simulink model "switching_controller_parallel_after_retraining"  (R2020a)
settings: Solver=FixedStepAuto  StartTime=0.0  StopTime=simulation.time_window  FixedStep=simulation.time_step  MaxStep=.2  RelTol=1e-3
model workspace (MAT data in the model file):
  PID_TRESH = 0.3
undefined symbols (not defined in the file): DiscIntNeverNeededParam
libraries: neural x72, simulink x1
(part 3 of 3)

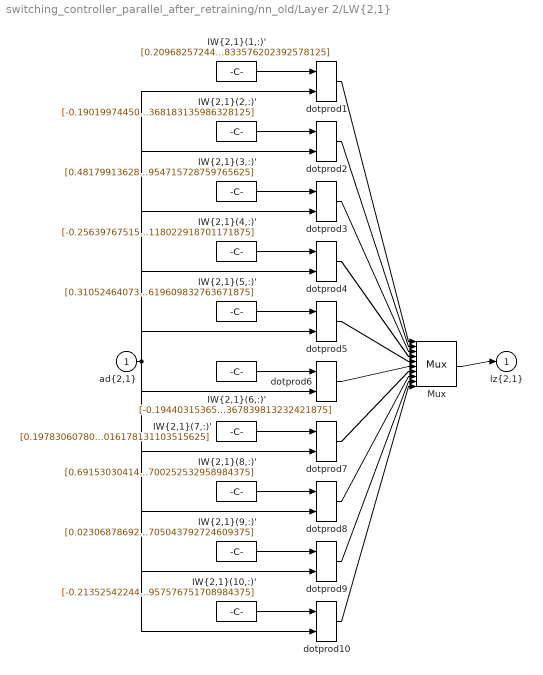
== system switching_controller_parallel_after_retraining/nn_old/Layer 2/LW{2,1} ==
  "ad{2,1}" : Inport  PortDimensions=20
      mask Display: e = 0.06;c1 = [120 230 180]/255;c2 = ([120 230 180]+0)/(256+128);c3 = ([120 230 180]+128)/(256+128);patch([0 1 1 0],[0 0 1 1],c1);patch([0 1 1 1-e 1-e 0+e],[0 0 1 1-e 0+e 0+e],c2);patch([0 0 1 1-e 0+e 0+e],[0 1 1 1-e 1-e 0+e],c3);plot([0 1 1 0 0],[0 0 1 1 0]);
  "IW{2,1}(1,:)'" : Constant  Value=[0.2096825724481717612146525198113522492349147796630859375;-0.0786324900654914726860766904792399145662784576416015625;-0.437914448078958240540003998830798082053661346435546875;0.1697961511740600226705311115438234992325305938720703125;0.55023489427883287561371616902761161327362060546875;-0.264125067565491977727987205071258358657360076904296875;-0.51948962376459417722429634522995911538600921630859375;0.332243447773037214876268308216822333633899688720703125;0.1565170256116675540081217832266702316701412200927734375;-0.63070597920798121549523784779012203216552734375;-0.27205863960363274589582260887254960834980010986328125;-0.1899107392996790821815267236161162145435810089111328125;-0.1897375152263709174871308960064197890460491180419921875;0.0256999070051998797226122661641056765802204608917236328125;0.309106789683368965437892939007724635303020477294921875;0.41159516280277974598078571943915449082851409912109375;0.394189668439436535773978675933904014527797698974609375;-0.58049288962487277654389572489890269935131072998046875;-0.3828300990267410330858410816290415823459625244140625;0.107169998780845709962505907242302782833576202392578125]
      mask Display: e = 0.06;c1 = [120 150 230]/255;c2 = ([120 150 230]+0)/383;c3 = ([120 150 230]+128)/383;patch([0 1 1 0],[0 0 1 1],c1);patch([0 1 1 1-e 1-e 0+e],[0 0 1 1-e 0+e 0+e],c2);patch([0 0 1 1-e 0+e 0+e],[0 1 1 1-e 1-e 0+e],c3);plot([0 1 1 0 0],[0 0 1 1 0]);disp('weights');
  "IW{2,1}(10,:)'" : Constant  Value=[-0.2135254224475679196704192008837708272039890289306640625;-0.46702854909986057929671687816153280436992645263671875;-0.491012465365010697393444161207298748195171356201171875;-0.56496432763406811972117793629877269268035888671875;-0.7227133704126142976775781789910979568958282470703125;0.170979606044271481568586068533477373421192169189453125;0.44374389503406319601452878487179987132549285888671875;0.0753589669229797476379673071278375573456287384033203125;-0.451293781769779134283027133278665132820606231689453125;0.0747381398083216963446062663933844305574893951416015625;-0.2762075487214932234536490796017460525035858154296875;-0.5460267148614048604571280520758591592311859130859375;0.0197077459717405478745178015742567367851734161376953125;-0.06834329138225274380413765129560488276183605194091796875;-0.1274719116559372700248076171192224137485027313232421875;-0.2139125442383393582712614033880527131259441375732421875;0.08760130810873280327033540970660396851599216461181640625;-0.10338035652578873857532215652099694125354290008544921875;0.2862039857027902645114636470680125057697296142578125;0.207128935024094518180248769567697308957576751708984375]
      mask Display: e = 0.06;c1 = [120 150 230]/255;c2 = ([120 150 230]+0)/383;c3 = ([120 150 230]+128)/383;patch([0 1 1 0],[0 0 1 1],c1);patch([0 1 1 1-e 1-e 0+e],[0 0 1 1-e 0+e 0+e],c2);patch([0 0 1 1-e 0+e 0+e],[0 1 1 1-e 1-e 0+e],c3);plot([0 1 1 0 0],[0 0 1 1 0]);disp('weights');
  "IW{2,1}(2,:)'" : Constant  Value=[-0.1901997445055658986223789952418883331120014190673828125;0.4889226492339562302191779963322915136814117431640625;0.5822125104488617974851649705669842660427093505859375;0.04192611403211977949556654721163795329630374908447265625;-0.068996957352157384235624704160727560520172119140625;-0.433158542617962993848124142459710128605365753173828125;-0.040131359594994149564417540432259556837379932403564453125;0.1937276670045855464508122167899273335933685302734375;0.452152014649461919670869747278629802167415618896484375;-0.55286960480626989866692611030885018408298492431640625;0.08355940035194704684773370217953925020992755889892578125;-0.1743526015010171958952156501254648901522159576416015625;0.11476795054229714521110139457960030995309352874755859375;-0.59479734978772358378051876570680178701877593994140625;0.276319293859086323461582423988147638738155364990234375;-0.10215476488676560051782615801130305044353008270263671875;-0.26107272028639816330297662716475315392017364501953125;-0.579920390991560896765122379292733967304229736328125;-0.1592627650723278665001458875849493779242038726806640625;-0.044346946533229077147542085413078893907368183135986328125]
      mask Display: e = 0.06;c1 = [120 150 230]/255;c2 = ([120 150 230]+0)/383;c3 = ([120 150 230]+128)/383;patch([0 1 1 0],[0 0 1 1],c1);patch([0 1 1 1-e 1-e 0+e],[0 0 1 1-e 0+e 0+e],c2);patch([0 0 1 1-e 0+e 0+e],[0 1 1 1-e 1-e 0+e],c3);plot([0 1 1 0 0],[0 0 1 1 0]);disp('weights');
  "IW{2,1}(3,:)'" : Constant  Value=[0.481799136287025364655534076518961228430271148681640625;0.387006958211107809919582223301404155790805816650390625;0.1919190370005954549004201226125587709248065948486328125;-0.43641483886599996555588631963473744690418243408203125;-0.49688357411208039504657563156797550618648529052734375;0.0020488012679514230364452576083067469880916178226470947265625;-0.184908572502721690877791616003378294408321380615234375;0.333455839511515084172543765816953964531421661376953125;-0.481036487364089826446189590569701977074146270751953125;0.34755666012205954640279514933354221284389495849609375;0.294843116199611898764487705193459987640380859375;0.2329942803063660139439861040955292992293834686279296875;-0.332425721969732690386223339373827911913394927978515625;-0.11204195263561367301718973976676352322101593017578125;-0.064344226389462966242405173034057952463626861572265625;-0.26447918257127212005030969521612860262393951416015625;-0.4404023331890851711278855873388238251209259033203125;-0.43485200204655460876068673314875923097133636474609375;0.4669108714352014910531352143152616918087005615234375;-0.387250838515266926354030374568537808954715728759765625]
      mask Display: e = 0.06;c1 = [120 150 230]/255;c2 = ([120 150 230]+0)/383;c3 = ([120 150 230]+128)/383;patch([0 1 1 0],[0 0 1 1],c1);patch([0 1 1 1-e 1-e 0+e],[0 0 1 1-e 0+e 0+e],c2);patch([0 0 1 1-e 0+e 0+e],[0 1 1 1-e 1-e 0+e],c3);plot([0 1 1 0 0],[0 0 1 1 0]);disp('weights');
  "IW{2,1}(4,:)'" : Constant  Value=[-0.25639767515399736197423408157192170619964599609375;-0.45921838490317312686528339327196590602397918701171875;-0.3293254038638953051787439108011312782764434814453125;-0.44158108947889973538991625900962390005588531494140625;0.233955749562186399170826689442037604749202728271484375;-0.027814737908238289232354389923784765414893627166748046875;-0.880326454366271438090052470215596258640289306640625;-0.1700238043081334915473945557096158154308795928955078125;-0.260201087444173750906628583834390155971050262451171875;0.52249104272064117449048126218258403241634368896484375;-0.045211937144701015711678593333999742753803730010986328125;0.056005248738155342935751690447432338260114192962646484375;0.0272144426463411977235029581834169221110641956329345703125;-0.55189260887602886729297324563958682119846343994140625;-0.2232599587265805818336872334839426912367343902587890625;-0.77589840738633253369727071913075633347034454345703125;-0.364528533738595894586609347243211232125759124755859375;-0.52690429597504129244356363415136002004146575927734375;0.2355191475436664294562660870724357664585113525390625;0.1088197708787270456820550634802202694118022918701171875]
      mask Display: e = 0.06;c1 = [120 150 230]/255;c2 = ([120 150 230]+0)/383;c3 = ([120 150 230]+128)/383;patch([0 1 1 0],[0 0 1 1],c1);patch([0 1 1 1-e 1-e 0+e],[0 0 1 1-e 0+e 0+e],c2);patch([0 0 1 1-e 0+e 0+e],[0 1 1 1-e 1-e 0+e],c3);plot([0 1 1 0 0],[0 0 1 1 0]);disp('weights');
  "IW{2,1}(5,:)'" : Constant  Value=[0.310524640737501023135536115660215727984905242919921875;0.0146429681645852023674780895134972524829208850860595703125;0.416071005130671578431389434626908041536808013916015625;0.2349476910365399240365746891257003881037235260009765625;0.0266711848666466681823106199544781702570617198944091796875;-0.2184710102237388540391549440755625255405902862548828125;2.094726675060243348269750640611164271831512451171875;-0.62331361106756000278750207144184969365596771240234375;-0.0203637098643958715238344581166529678739607334136962890625;-0.0271757616677543722971677198074758052825927734375;-0.099119675867250067735625407294719479978084564208984375;0.12043446514574361605465213642673916183412075042724609375;-0.88670130489474974222474656926351599395275115966796875;0.25211544537308194779967607246362604200839996337890625;-0.11259143114996773837876986590345040895044803619384765625;0.61060143798205601672890452391584403812885284423828125;-0.452607547304984703107066934535396285355091094970703125;-0.373800814753432908421615366023615933954715728759765625;-0.0172484013592278662141410450203693471848964691162109375;0.5859028956126166587381476347218267619609832763671875]
      mask Display: e = 0.06;c1 = [120 150 230]/255;c2 = ([120 150 230]+0)/383;c3 = ([120 150 230]+128)/383;patch([0 1 1 0],[0 0 1 1],c1);patch([0 1 1 1-e 1-e 0+e],[0 0 1 1-e 0+e 0+e],c2);patch([0 0 1 1-e 0+e 0+e],[0 1 1 1-e 1-e 0+e],c3);plot([0 1 1 0 0],[0 0 1 1 0]);disp('weights');
  "IW{2,1}(6,:)'" : Constant  Value=[-0.1944031536556706518670267769266502000391483306884765625;-0.295446194500971426322166735189966857433319091796875;-0.54770988104943951757519471357227303087711334228515625;-0.404408826705410950896890653893933631479740142822265625;-0.83869791765557566431965597075759433209896087646484375;-0.325816969167355974246191863130661658942699432373046875;-0.2072529611842870156390716829264420084655284881591796875;0.240744674786417700573792899376712739467620849609375;-0.1674498692919050568672645340484450571238994598388671875;-0.28891816291228311630590042113908566534519195556640625;-0.22131051344031948957535860245116055011749267578125;-0.10913280135527003711359839144279249012470245361328125;-0.4918651471215065296149759888066910207271575927734375;0.240001755562789742537432857716339640319347381591796875;0.6937710080396275458269883529283106327056884765625;0.06323702674474794560577350921448669396340847015380859375;-0.2752337038543775094012744375504553318023681640625;-0.255069800974772997737005653107189573347568511962890625;-0.285682618796993192944455586257390677928924560546875;-0.31188153451426436912896633657510392367839813232421875]
      mask Display: e = 0.06;c1 = [120 150 230]/255;c2 = ([120 150 230]+0)/383;c3 = ([120 150 230]+128)/383;patch([0 1 1 0],[0 0 1 1],c1);patch([0 1 1 1-e 1-e 0+e],[0 0 1 1-e 0+e 0+e],c2);patch([0 0 1 1-e 0+e 0+e],[0 1 1 1-e 1-e 0+e],c3);plot([0 1 1 0 0],[0 0 1 1 0]);disp('weights');
  "IW{2,1}(7,:)'" : Constant  Value=[0.1978306078065260875664677087115705944597721099853515625;-0.59250058903084179551257193452329374849796295166015625;0.64639267817649359582077295272029004991054534912109375;-0.53285927855746084702559528523124754428863525390625;0.588817119499761343348609443637542426586151123046875;-0.348911668719428025298157081124372780323028564453125;-0.64457560060689800263133975022356025874614715576171875;0.0562679680258353076549582283405470661818981170654296875;0.5623436544941402548403175387647934257984161376953125;0.1281096810622278925340111754849203862249851226806640625;0.161634591264916249730987374277901835739612579345703125;-0.313017483079470526519116901909001171588897705078125;0.38128996525822411722828064739587716758251190185546875;-0.1756877707290915580085055580639163963496685028076171875;-0.380091610378465116770740905849379487335681915283203125;-0.1356942844701036487986556267060223035514354705810546875;0.1185198788428162564034806791823939420282840728759765625;-0.254421588692579081492084469573455862700939178466796875;-0.2881679500781364478001478346413932740688323974609375;-0.2391992576729999042672858422520221211016178131103515625]
      mask Display: e = 0.06;c1 = [120 150 230]/255;c2 = ([120 150 230]+0)/383;c3 = ([120 150 230]+128)/383;patch([0 1 1 0],[0 0 1 1],c1);patch([0 1 1 1-e 1-e 0+e],[0 0 1 1-e 0+e 0+e],c2);patch([0 0 1 1-e 0+e 0+e],[0 1 1 1-e 1-e 0+e],c3);plot([0 1 1 0 0],[0 0 1 1 0]);disp('weights');
  "IW{2,1}(8,:)'" : Constant  Value=[0.6915303041485005852706535733886994421482086181640625;-0.013943214076003206114418020433731726370751857757568359375;0.197633492735798832473648189989035017788410186767578125;-0.1829294585786688520645526523367152549326419830322265625;0.41194460235457064367636803581262938678264617919921875;0.2697850457965962345241450748289935290813446044921875;0.2278285465289087985407689984640455804765224456787109375;-0.594187771563595479307196001172997057437896728515625;0.33636923738323110111281266654259525239467620849609375;-0.10886422192579021939184968914560158737003803253173828125;0.330016039728184329415938691454357467591762542724609375;-0.5612454717224470979175521279103122651576995849609375;-0.5208533730307125519942701430409215390682220458984375;0.0927595999828694228739323079935275018215179443359375;-0.295470908532163789583790958204190246760845184326171875;0.2464488470485728111025736097872140817344188690185546875;-0.253925461039385014228031423044740222394466400146484375;-0.44676839807914936475441436414257623255252838134765625;-0.343537111312336163049252490964136086404323577880859375;0.04503529300945828539592952211023657582700252532958984375]
      mask Display: e = 0.06;c1 = [120 150 230]/255;c2 = ([120 150 230]+0)/383;c3 = ([120 150 230]+128)/383;patch([0 1 1 0],[0 0 1 1],c1);patch([0 1 1 1-e 1-e 0+e],[0 0 1 1-e 0+e 0+e],c2);patch([0 0 1 1-e 0+e 0+e],[0 1 1 1-e 1-e 0+e],c3);plot([0 1 1 0 0],[0 0 1 1 0]);disp('weights');
  "IW{2,1}(9,:)'" : Constant  Value=[0.0230687869274933711472019837174229905940592288970947265625;0.063142758058253922737179664181894622743129730224609375;0.15173098751753089086236059301882050931453704833984375;0.00443276217291526698771608749893857748247683048248291015625;0.3879819604221512729935739116626791656017303466796875;0.67423681207509444934800058035762049257755279541015625;-0.10965154605191219927551316004610271193087100982666015625;0.54284957310125514506893296129419468343257904052734375;0.485695834032557727244494572005351074039936065673828125;-0.3061948412592043755608983701677061617374420166015625;0.359525507608165872941441421062336303293704986572265625;0.60766075733581847995168345732963643968105316162109375;-0.1918328188570195547146823855655384249985218048095703125;0.56745984668721305421712486349861137568950653076171875;0.392602621322820033444855880588875152170658111572265625;-0.534358634420198708170346435508690774440765380859375;0.023661369862847399236915890696764108724892139434814453125;-0.1696865058591041364177698369530844502151012420654296875;0.4660595474214745959073979975073598325252532958984375;-0.439829607094486652041354091124958358705043792724609375]
      mask Display: e = 0.06;c1 = [120 150 230]/255;c2 = ([120 150 230]+0)/383;c3 = ([120 150 230]+128)/383;patch([0 1 1 0],[0 0 1 1],c1);patch([0 1 1 1-e 1-e 0+e],[0 0 1 1-e 0+e 0+e],c2);patch([0 0 1 1-e 0+e 0+e],[0 1 1 1-e 1-e 0+e],c3);plot([0 1 1 0 0],[0 0 1 1 0]);disp('weights');
  Mux : Mux  Inputs=10
      mask Display: e = 0.06;c1 = [120 150 230]/255;c2 = ([120 150 230]+0)/383;c3 = ([120 150 230]+128)/383;patch([0 1 1 0],[0 0 1 1],c1);patch([0 1 1 1-e 1-e 0+e],[0 0 1 1-e 0+e 0+e],c2);patch([0 0 1 1-e 0+e 0+e],[0 1 1 1-e 1-e 0+e],c3);plot([0 1 1 0 0],[0 0 1 1 0]);disp('Mux');
  dotprod{1..10} (10 alike) : neural/Weight Functions/dotprod
  "lz{2,1}" : Outport
      mask Display: e = 0.06;c1 = [120 230 180]/255;c2 = ([120 230 180]+0)/(256+128);c3 = ([120 230 180]+128)/(256+128);patch([0 1 1 0],[0 0 1 1],c1);patch([0 1 1 1-e 1-e 0+e],[0 0 1 1-e 0+e 0+e],c2);patch([0 0 1 1-e 0+e 0+e],[0 1 1 1-e 1-e 0+e],c3);plot([0 1 1 0 0],[0 0 1 1 0]);
  wires:
  "IW{2,1}(1,:)'"/1 -> dotprod1/1
  "ad{2,1}"/1 -> dotprod1/2, dotprod2/2, dotprod3/2, dotprod4/2, dotprod5/2, dotprod6/2, dotprod7/2, dotprod8/2, dotprod9/2, dotprod10/2
  dotprod1/1 -> Mux/1
  "IW{2,1}(2,:)'"/1 -> dotprod2/1
  dotprod2/1 -> Mux/2
  "IW{2,1}(3,:)'"/1 -> dotprod3/1
  dotprod3/1 -> Mux/3
  "IW{2,1}(4,:)'"/1 -> dotprod4/1
  dotprod4/1 -> Mux/4
  "IW{2,1}(5,:)'"/1 -> dotprod5/1
  dotprod5/1 -> Mux/5
  "IW{2,1}(6,:)'"/1 -> dotprod6/1
  dotprod6/1 -> Mux/6
  "IW{2,1}(7,:)'"/1 -> dotprod7/1
  dotprod7/1 -> Mux/7
  "IW{2,1}(8,:)'"/1 -> dotprod8/1
  dotprod8/1 -> Mux/8
  "IW{2,1}(9,:)'"/1 -> dotprod9/1
  dotprod9/1 -> Mux/9
  "IW{2,1}(10,:)'"/1 -> dotprod10/1
  dotprod10/1 -> Mux/10
  Mux/1 -> "lz{2,1}"/1

== system switching_controller_parallel_after_retraining/nn_old/Layer 3/Delays 1 ==
  "p{3}" : Inport  PortDimensions=10
      mask Display: e = 0.06;c1 = [120 230 180]/255;c2 = ([120 230 180]+0)/(256+128);c3 = ([120 230 180]+128)/(256+128);patch([0 1 1 0],[0 0 1 1],c1);patch([0 1 1 1-e 1-e 0+e],[0 0 1 1-e 0+e 0+e],c2);patch([0 0 1 1-e 0+e 0+e],[0 1 1 1-e 1-e 0+e],c3);plot([0 1 1 0 0],[0 0 1 1 0]);
  mux : Mux  Inputs=1
      mask Display: e = 0.06;c1 = [120 150 230]/255;c2 = ([120 150 230]+0)/383;c3 = ([120 150 230]+128)/383;patch([0 1 1 0],[0 0 1 1],c1);patch([0 1 1 1-e 1-e 0+e],[0 0 1 1-e 0+e 0+e],c2);patch([0 0 1 1-e 0+e 0+e],[0 1 1 1-e 1-e 0+e],c3);plot([0 1 1 0 0],[0 0 1 1 0]);disp('Mux')
  "pd{3,2}" : Outport
      mask Display: e = 0.06;c1 = [120 230 180]/255;c2 = ([120 230 180]+0)/(256+128);c3 = ([120 230 180]+128)/(256+128);patch([0 1 1 0],[0 0 1 1],c1);patch([0 1 1 1-e 1-e 0+e],[0 0 1 1-e 0+e 0+e],c2);patch([0 0 1 1-e 0+e 0+e],[0 1 1 1-e 1-e 0+e],c3);plot([0 1 1 0 0],[0 0 1 1 0]);
  wires:
  "p{3}"/1 -> mux/1
  mux/1 -> "pd{3,2}"/1

== system switching_controller_parallel_after_retraining/nn_old/Layer 3/LW{3,2} ==
  "ad{3,2}" : Inport  PortDimensions=10
      mask Display: e = 0.06;c1 = [120 230 180]/255;c2 = ([120 230 180]+0)/(256+128);c3 = ([120 230 180]+128)/(256+128);patch([0 1 1 0],[0 0 1 1],c1);patch([0 1 1 1-e 1-e 0+e],[0 0 1 1-e 0+e 0+e],c2);patch([0 0 1 1-e 0+e 0+e],[0 1 1 1-e 1-e 0+e],c3);plot([0 1 1 0 0],[0 0 1 1 0]);
  "IW{3,2}(1,:)'" : Constant  Value=[-0.0183091459994614534634305158533607027493417263031005859375;0.7708433750167789089147163394954986870288848876953125;-0.0026554652690759452011992625131142631289549171924591064453125;0.82194094287886476646320943473256193101406097412109375;-1.5258437616277029658107267096056602895259857177734375;-0.2304305859716547499882466354392818175256252288818359375;-0.798920136160017335669181193225085735321044921875;0.5765448253543394852016490403912030160427093505859375;0.84849162700978164597387376488768495619297027587890625;-0.36467299153547971801714311368414200842380523681640625]
      mask Display: e = 0.06;c1 = [120 150 230]/255;c2 = ([120 150 230]+0)/383;c3 = ([120 150 230]+128)/383;patch([0 1 1 0],[0 0 1 1],c1);patch([0 1 1 1-e 1-e 0+e],[0 0 1 1-e 0+e 0+e],c2);patch([0 0 1 1-e 0+e 0+e],[0 1 1 1-e 1-e 0+e],c3);plot([0 1 1 0 0],[0 0 1 1 0]);disp('weights');
  Mux : Mux  Inputs=1
      mask Display: e = 0.06;c1 = [120 150 230]/255;c2 = ([120 150 230]+0)/383;c3 = ([120 150 230]+128)/383;patch([0 1 1 0],[0 0 1 1],c1);patch([0 1 1 1-e 1-e 0+e],[0 0 1 1-e 0+e 0+e],c2);patch([0 0 1 1-e 0+e 0+e],[0 1 1 1-e 1-e 0+e],c3);plot([0 1 1 0 0],[0 0 1 1 0]);disp('Mux');
  dotprod1 : neural/Weight Functions/dotprod
  "lz{3,2}" : Outport
      mask Display: e = 0.06;c1 = [120 230 180]/255;c2 = ([120 230 180]+0)/(256+128);c3 = ([120 230 180]+128)/(256+128);patch([0 1 1 0],[0 0 1 1],c1);patch([0 1 1 1-e 1-e 0+e],[0 0 1 1-e 0+e 0+e],c2);patch([0 0 1 1-e 0+e 0+e],[0 1 1 1-e 1-e 0+e],c3);plot([0 1 1 0 0],[0 0 1 1 0]);
  wires:
  "IW{3,2}(1,:)'"/1 -> dotprod1/1
  "ad{3,2}"/1 -> dotprod1/2
  dotprod1/1 -> Mux/1
  Mux/1 -> "lz{3,2}"/1

== stateflow chart switching_controller_parallel_after_retraining/SwitchingController ==
  state STEADY
    entry: u = 0;
  state P
    du:
    u = p_control(e);
    state u = p_control(e) [function]
  state PID
    du:
    u = pid_control(e);
    state u = pid_control(e) [function]
  (default) -> STEADY
  STEADY -> P : [e > -0.01]
  P -> PID : [e < PID_TRESH]
  data: e function_input; u function_output; e function_input; u function_output; e input; u output double; PID output boolean; PID_TRESH parameter; P output boolean
